simulink model "sim_Rectification"  (Simulink 7.9)
settings: Solver=ode3  StartTime=0.0  StopTime=0.1  RelTol=1e-3
libraries: powerlib x23
settings Model: Creator=Kun Zhang  LastModifiedBy=LYN
settings DebuggingCC: FcnCallInpInsideContextMsg=Use local settings
settings GRTTargetCC: CombineOutputUpdateFcns=off  GRTInterface=on

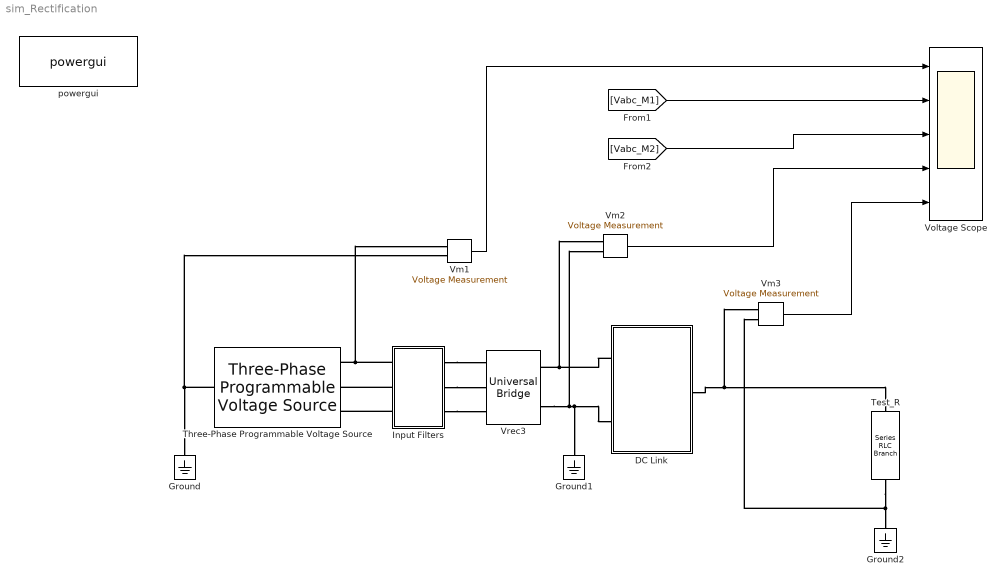
== system sim_Rectification ==
  DC Link : Subsystem
      mask Display:
      | port_label('lconn',1,'IN')
      | port_label('lconn',2,'GND')
      | port_label('rconn',1,'OUT')
  Ground : powerlib/Elements/Ground  LConnTagsString=a
  Ground1 : powerlib/Elements/Ground  LConnTagsString=a
  Ground2 : powerlib/Elements/Ground  LConnTagsString=a
  Input Filters : Subsystem
  Test_R : powerlib/Elements/Series RLC Branch  LConnTagsString=__new0  RConnTagsString=__new0  BranchType=R  Resistance=100  Inductance=1e-3  SetiL0=off  InitialCurrent=0  Capacitance=1e-6  Setx0=off  InitialVoltage=0  Measurements=None
  Three-Phase Programmable Voltage Source : powerlib/Electrical Sources/Three-Phase Programmable Voltage Source  PositiveSequence=[220 0 50]  VariationEntity=None  VariationType=Step  VariationTypeAlt=Step  VariationStep=0.5  VariationRate=10  VariationMagnitude=0.3  VariationFrequency=2  VariationTiming=[1 2]  VariationPhaseA=off  Amplitudes=[1 0.8 1.2 1.0]  TimeValues=[0 0.1 0.15 0.2]  HarmonicGeneration=on  HarmonicA=[3 0.05 0 0]  HarmonicB=[13 0.05 0 0]  Timing="[0  0.5]"  BusType=swing  Pref=0  Qref=0  Qmin=-inf  Qmax=inf
  Vm1 : powerlib/Measurements/Voltage Measurement  PhasorSimulation=off  OutputType=Complex  PSBequivalent=0
  Vm2 : powerlib/Measurements/Voltage Measurement  PhasorSimulation=off  OutputType=Complex  PSBequivalent=0
  Vm3 : powerlib/Measurements/Voltage Measurement  PhasorSimulation=off  OutputType=Complex  PSBequivalent=0
  Voltage Scope : Scope  NumInputPorts=5
      settings: TimeRange=0.02  YMin=-100~-200~-100~0~0  YMax=100~100~100~100~100  SaveName=sim_Rectification
  Vrec3 : powerlib/Power Electronics/Universal Bridge  Arms=3  SnubberResistance=500  SnubberCapacitance=1.0e-007  Device=Diodes  Ron=1e-3  Lon=0  ForwardVoltages="[  0  0  ]"  ForwardVoltage=0  GTOparameters=[ 10e-6 , 20e-6 ]  IGBTparameters=[ 1e-6 , 2e-6 ]  Measurements=None  Measurements_2=None  converterType=Rectifier
  powergui : powerlib/powergui  Priority=1  SimulationMode=Discrete  SolverType=Tustin  SampleTime=1e-6  frequency=60  SPID=off  DisableSnubberDevices=off  DisableRonSwitches=off  DisableVfSwitches=off  SwTol=0  Interpol=off  DisplayEquations=off  FunctionMessages=off  frequencyindice=50  Pbase=100e6  ErrMax=1e-4  Iterations=50  UnitsV=kV  UnitsW=MW  echomessages=off  HookPort=off  EnableUseOfTLC=off  x0status=blocks  RestoreLinks=warning  ResistiveCurrentMeasurement=off  Ylog=off  Xlog=on  ShowGrid=off  save=off  variable=ZData  structure=sim_Rectification  ZoomFFT=off  StartTime=0  cycles=4  DisplayStyle=1  fundamental=50  FreqAxis=off  MaxFrequency=1000  frequencyindicesteady=1  display=off  methode=off
  wires:
  Vm1/1 -> Voltage Scope/1
  [Vabc_M1] -> Voltage Scope/2
  Vm3/1 -> Voltage Scope/5
  Vm2/1 -> Voltage Scope/4
  [Vabc_M2] -> Voltage Scope/3
  connections:
  Vrec3/RConn2 -- Ground1/LConn1 -- DC Link/LConn2 -- Vm2/LConn2
  DC Link/RConn1 -- Test_R/LConn1 -- Vm3/LConn1
  Three-Phase Programmable Voltage Source/LConn1 -- Ground/LConn1 -- Vm1/LConn2
  DC Link/LConn1 -- Vrec3/RConn1 -- Vm2/LConn1
  Input Filters/LConn1 -- Three-Phase Programmable Voltage Source/RConn1 -- Vm1/LConn1
  Test_R/RConn1 -- Ground2/LConn1 -- Vm3/LConn2
  Input Filters/RConn1 -- Vrec3/LConn1
  Input Filters/RConn2 -- Vrec3/LConn2
  Input Filters/RConn3 -- Vrec3/LConn3
  Input Filters/LConn2 -- Three-Phase Programmable Voltage Source/RConn2
  Input Filters/LConn3 -- Three-Phase Programmable Voltage Source/RConn3

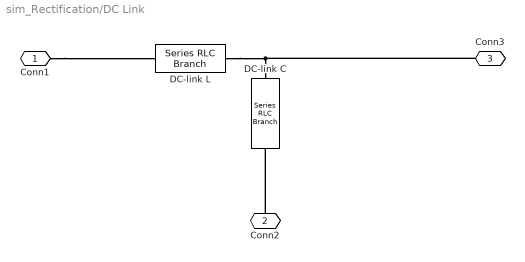
== system sim_Rectification/DC Link ==
  DC-link C : powerlib/Elements/Series RLC Branch  LConnTagsString=__new0  RConnTagsString=__new0  BranchType=C  Resistance=1  Inductance=1e-3  SetiL0=off  InitialCurrent=0  Capacitance=5000e-6  Setx0=off  InitialVoltage=0  Measurements=None
  DC-link L : powerlib/Elements/Series RLC Branch  LConnTagsString=__new0  RConnTagsString=__new0  BranchType=L  Resistance=1  Inductance=200e-6  SetiL0=off  InitialCurrent=0  Capacitance=1e-6  Setx0=off  InitialVoltage=0  Measurements=Branch voltage and current
  Conn1 : PMIOPort  Port=1  Side=Left
  Conn2 : PMIOPort  Port=2  Side=Left
  Conn3 : PMIOPort  Port=3  Side=Right
  connections:
  DC-link L/RConn1 -- DC-link C/LConn1 -- Conn3/RConn1
  Conn1/RConn1 -- DC-link L/LConn1
  Conn2/RConn1 -- DC-link C/RConn1

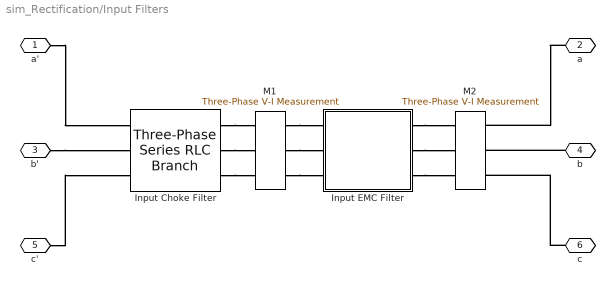
== system sim_Rectification/Input Filters ==
  Input Choke Filter : powerlib/Elements/Three-Phase Series RLC Branch  LConnTagsString=A|B|C  RConnTagsString=A|B|C  BranchType=RL  Resistance=1.0  Inductance=1e-5  Capacitance=1e-6  Measurements=None
  Input EMC Filter : Subsystem
  M1 : powerlib/Measurements/Three-Phase V-I Measurement  VoltageMeasurement=phase-to-phase  SetLabelV=on  LabelV=Vabc_M1  Vpu=off  VpuLL=off  CurrentMeasurement=yes  SetLabelI=on  LabelI=Iabc_M1  Ipu=off  Pbase=100e6  Vbase=500e3  OutputType=Complex  PhasorSimulation=off  PSBequivalent=0
  M2 : powerlib/Measurements/Three-Phase V-I Measurement  VoltageMeasurement=phase-to-phase  SetLabelV=on  LabelV=Vabc_M2  Vpu=off  VpuLL=off  CurrentMeasurement=yes  SetLabelI=on  LabelI=Iabc_M2  Ipu=off  Pbase=100e6  Vbase=500e3  OutputType=Complex  PhasorSimulation=off  PSBequivalent=0
  " a'" : PMIOPort  Port=1  Side=Left
  a : PMIOPort  Port=2  Side=Right
  b' : PMIOPort  Port=3  Side=Left
  b : PMIOPort  Port=4  Side=Right
  c' : PMIOPort  Port=5  Side=Left
  c : PMIOPort  Port=6  Side=Right
  connections:
  Input Choke Filter/RConn1 -- M1/LConn1
  Input Choke Filter/RConn2 -- M1/LConn2
  Input Choke Filter/RConn3 -- M1/LConn3
  M1/RConn1 -- Input EMC Filter/LConn1
  M1/RConn2 -- Input EMC Filter/LConn2
  M1/RConn3 -- Input EMC Filter/LConn3
  Input EMC Filter/RConn1 -- M2/LConn1
  Input EMC Filter/RConn2 -- M2/LConn2
  Input EMC Filter/RConn3 -- M2/LConn3
  " a'"/RConn1 -- Input Choke Filter/LConn1
  a/RConn1 -- M2/RConn1
  b'/RConn1 -- Input Choke Filter/LConn2
  b/RConn1 -- M2/RConn2
  c'/RConn1 -- Input Choke Filter/LConn3
  c/RConn1 -- M2/RConn3

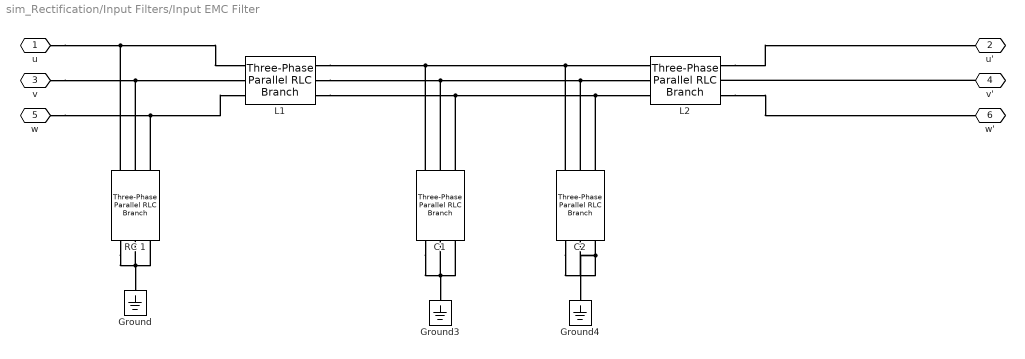
== system sim_Rectification/Input Filters/Input EMC Filter ==
  C1 : powerlib/Elements/Three-Phase Parallel RLC Branch  LConnTagsString=A|B|C  RConnTagsString=A|B|C  BranchType=C  Resistance=1.5e6  Inductance=0.15e-5  Capacitance=0.47e-6  Measurements=None
  C2 : powerlib/Elements/Three-Phase Parallel RLC Branch  LConnTagsString=A|B|C  RConnTagsString=A|B|C  BranchType=C  Resistance=1.5e6  Inductance=0.15e-5  Capacitance=20e-9  Measurements=None
  Ground : powerlib/Elements/Ground  LConnTagsString=a
  Ground3 : powerlib/Elements/Ground  LConnTagsString=a
  Ground4 : powerlib/Elements/Ground  LConnTagsString=a
  L1 : powerlib/Elements/Three-Phase Parallel RLC Branch  LConnTagsString=A|B|C  RConnTagsString=A|B|C  BranchType=L  Resistance=1  Inductance=0.15e-3  Capacitance=1e-6  Measurements=None
  L2 : powerlib/Elements/Three-Phase Parallel RLC Branch  LConnTagsString=A|B|C  RConnTagsString=A|B|C  BranchType=L  Resistance=1  Inductance=0.15e-4  Capacitance=1e-6  Measurements=None
  RC 1 : powerlib/Elements/Three-Phase Parallel RLC Branch  LConnTagsString=A|B|C  RConnTagsString=A|B|C  BranchType=RC  Resistance=1.5e6  Inductance=0.15e-5  Capacitance=0.47e-6  Measurements=None
  u : PMIOPort  Port=1  Side=Left
  u' : PMIOPort  Port=2  Side=Right
  v : PMIOPort  Port=3  Side=Left
  v' : PMIOPort  Port=4  Side=Right
  w : PMIOPort  Port=5  Side=Left
  w' : PMIOPort  Port=6  Side=Right
  connections:
  u/RConn1 -- L1/LConn1 -- RC 1/RConn1
  L2/RConn1 -- u'/RConn1
  v/RConn1 -- L1/LConn2 -- RC 1/RConn2
  L1/RConn2 -- C1/RConn2 -- L2/LConn2 -- C2/RConn2
  v'/RConn1 -- L2/RConn2
  w/RConn1 -- L1/LConn3 -- RC 1/RConn3
  L2/RConn3 -- w'/RConn1
  RC 1/LConn1 -- Ground/LConn1 -- RC 1/LConn2 -- RC 1/LConn3
  C1/LConn1 -- Ground3/LConn1 -- C1/LConn3 -- C1/LConn2
  L1/RConn3 -- C1/RConn3 -- L2/LConn3 -- C2/RConn3
  L1/RConn1 -- C1/RConn1 -- L2/LConn1 -- C2/RConn1
  C2/LConn3 -- Ground4/LConn1 -- C2/LConn1 -- C2/LConn2
